simulink model "E020_B2_ton_boost_from_ideal_iqcot_20260629"  (R2024b)
settings: Solver=VariableStepAuto  StartTime=0.0  StopTime=0.54e-3  MaxStep=5e-9  RelTol=1e-3
undefined symbols (not defined in the file): A_init, A_lower, A_upper, Cout, DCR_L1, DCR_L2, DCR_L3, DCR_L4, E020_Boost_Decay_Rate, E020_CurrentLimit_Guard, E020_TonBoost_Enable, E020_TonBoost_Window, E020_Undershoot_Band, E020_Vref, ESR_C, IdealIQCOT_Enable, IL_adc_counts_per_A, IL_pk_limit_adc_neg, IL_pk_limit_adc_pos, Iload_final, Iload_initial, Iph, Iqcot_enable, kappa_cmd, Kiqcot, Kvc_iqcot, L, Lambda0_iqcot, Lambda_m2, rho_cmd, Ri_iqcot, t_load_step, Tblank, Tdead, Tiqcot_leak, Toff_min, Ton_cmd, Ton_iq_max, Ton_iq_min, Ts_ctrl, Tslot, Tss, Tton_boost_max, Vc_bias_iqcot, Vcot_ramp_amp, Vcot_ramp_enable, Vhys, Vin, Vo_ref
libraries: simulink x29, spsCurrentMeasurementLib x8, spsMosfetLib x8, spsSeriesRLCBranchLib x5, spsVoltageMeasurementLib x5, spsDCVoltageSourceLib x4, spsControlledCurrentSourceLib x1, spsGroundLib x1, spspowerguiLib x1
(part 2 of 2)

== matlab function E020_B2_ton_boost_from_ideal_iqcot_20260629/Ideal_Digital_IQCOT_Request/IQCOT_Event_Core ==
  data: e_v input double size=1; REQ_iqcot output double size=1; IL1 input double size=1; IL2 input double size=1; IL3 input double size=1; IL4 input double size=1; phase_idx input double size=1; tr_reset input double size=1; enable input double size=1; Ts_ctrl_in input double size=1; Lambda0_in input double size=1; Lambda_m2_in input double size=1; rho_cmd_in input double size=1; Ri_in input double size=1; Kvc_in input double size=1; Vc_bias_in input double size=1; kappa_cmd_in input double size=1; A_init_in input double size=1; A_lower_in input double size=1; A_upper_in input double size=1; A_iqcot output double size=1; Lambda_i output double size=1; h_iqcot output double size=1; IL_sel output double size=1; vc_ctrl output double size=1
function [REQ_iqcot,A_iqcot,Lambda_i,h_iqcot,IL_sel,vc_ctrl] = IQCOT_Event_Core(e_v,IL1,IL2,IL3,IL4,phase_idx,tr_reset,enable,Ts_ctrl_in,Lambda0_in,Lambda_m2_in,rho_cmd_in,Ri_in,Kvc_in,Vc_bias_in,kappa_cmd_in,A_init_in,A_lower_in,A_upper_in)
%#codegen
REQ_iqcot = 0.0;
A_iqcot = 0.0;
Lambda_i = 0.0;
h_iqcot = 0.0;
IL_sel = 0.0;
vc_ctrl = 0.0;
persistent Astate reset_prev phase_prev
if isempty(Astate)
    Astate = double(A_init_in);
end
if isempty(reset_prev)
    reset_prev = 0.0;
end
if isempty(phase_prev)
    phase_prev = 0.0;
end
p = floor(double(phase_idx));
p = mod(p, 4);
if p == 0
    IL_sel = IL1;
elseif p == 1
    IL_sel = IL2;
elseif p == 2
    IL_sel = IL3;
else
    IL_sel = IL4;
end
Ri_eff = Ri_in * exp(kappa_cmd_in);
vc_ctrl = Vc_bias_in + Kvc_in * e_v;
h_iqcot = vc_ctrl - Ri_eff * IL_sel;
Lambda_i = Lambda0_in * (1 + rho_cmd_in) + Lambda_m2_in * cos(pi * p);
if Lambda_i < eps
    Lambda_i = eps;
end
A_update = Astate + Ts_ctrl_in * h_iqcot;
if A_update < A_lower_in
    A_update = A_lower_in;
end
if A_update > A_upper_in
    A_update = A_upper_in;
end
REQ_iqcot = double((enable > 0.5) && (A_update >= Lambda_i));
A_iqcot = A_update;
reset_rise = (tr_reset > 0.5) && (reset_prev <= 0.5);
phase_change = (p ~= phase_prev);
if enable <= 0.5
    Astate = A_init_in;
elseif reset_rise || phase_change
    Astate = A_init_in;
else
    Astate = A_update;
end
reset_prev = double(tr_reset);
phase_prev = p;

== matlab function E020_B2_ton_boost_from_ideal_iqcot_20260629/E020_TonBoost2 ==
  data: ton_in input double size=1; ton_out output double size=1; t input double size=1; t_step input double size=1; t_window input double size=1; t_max input double size=1; decay_rate input double size=1; enable input double size=1; vout input double size=1; vref input double size=1; band input double size=1; il_i input double size=1; current_limit input double size=1; boost_active output double size=1
function [ton_out,boost_active] = ton_boost(ton_in,t,t_step,t_window,t_max,decay_rate,enable,vout,vref,band,il_i,current_limit)
%#codegen
age = t - t_step;
in_window = (enable > 0.5) && (age >= 0.0) && (age <= t_window);
deficit = vout <= (vref - band);
guard_ok = (current_limit <= 0.0) || (abs(il_i) <= current_limit);
active = in_window && deficit && guard_ok && (t_max > ton_in);
if active
    decay = exp(-max(decay_rate, 0.0) * max(age, 0.0));
    target = ton_in + (t_max - ton_in) * decay;
    ton_out = min(max(target, ton_in), t_max);
else
    ton_out = ton_in;
end
boost_active = double(active);

== matlab function E020_B2_ton_boost_from_ideal_iqcot_20260629/E020_TonBoost3 ==
  data: ton_in input double size=1; ton_out output double size=1; t input double size=1; t_step input double size=1; t_window input double size=1; t_max input double size=1; decay_rate input double size=1; enable input double size=1; vout input double size=1; vref input double size=1; band input double size=1; il_i input double size=1; current_limit input double size=1; boost_active output double size=1
function [ton_out,boost_active] = ton_boost(ton_in,t,t_step,t_window,t_max,decay_rate,enable,vout,vref,band,il_i,current_limit)
%#codegen
age = t - t_step;
in_window = (enable > 0.5) && (age >= 0.0) && (age <= t_window);
deficit = vout <= (vref - band);
guard_ok = (current_limit <= 0.0) || (abs(il_i) <= current_limit);
active = in_window && deficit && guard_ok && (t_max > ton_in);
if active
    decay = exp(-max(decay_rate, 0.0) * max(age, 0.0));
    target = ton_in + (t_max - ton_in) * decay;
    ton_out = min(max(target, ton_in), t_max);
else
    ton_out = ton_in;
end
boost_active = double(active);
